simulink model "gm_sampleModel1902_sub_sub"  (R2023a)
settings: Solver=VariableStepAuto  StartTime=0.0  StopTime=10.0  RelTol=1e-3
libraries: hdlsllib x4, simulink x1
settings Model: Creator=user1  LastModifiedBy=user1
settings OptimizationCC: BlockReduction=off  ConditionallyExecuteInputs=off
settings DebuggingCC: InheritedTsInSrcMsg=none

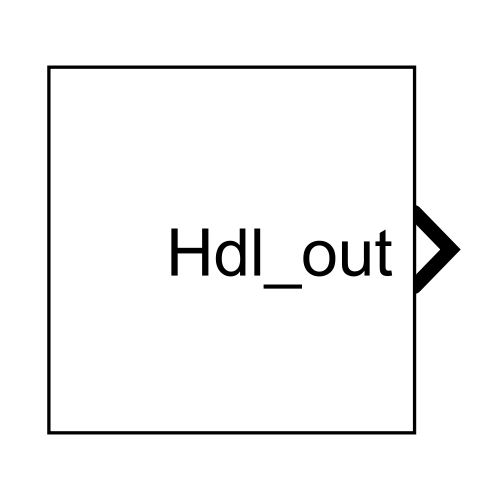
[thumbnail: Simulink's stored preview of the top-level diagram]
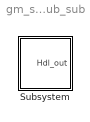
== system gm_sampleModel1902_sub_sub ==
  Subsystem : Subsystem

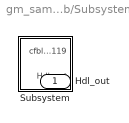
== system gm_sampleModel1902_sub_sub/Subsystem ==
  Subsystem : Subsystem
  Hdl_out : Outport  OutDataTypeStr=uint8

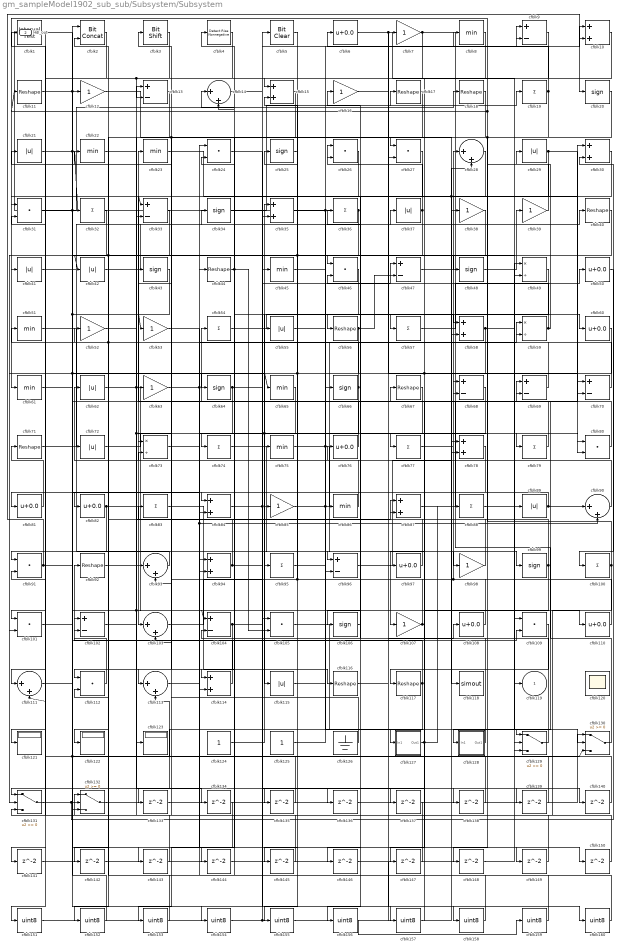
== system gm_sampleModel1902_sub_sub/Subsystem/Subsystem ==
  cfblk1 : hdlsllib/Logic and Bit Operations/Interval Test  IntervalClosedRight=on  uplimit=0.5  IntervalClosedLeft=on  lowlimit=-0.5  OutDataTypeStr=uint8
  cfblk{10,15,30,35,58,78,84,87,94,114} (10 alike) : Sum  OutDataTypeStr=uint8
  cfblk{19,32,36,54,57,74,77,79,83,88,95,100} (12 alike) : Sum  Inputs=+  OutDataTypeStr=uint8
  cfblk{24,26..27,31,46,80,91,101,105,109,112} (11 alike) : DotProduct  OutDataTypeStr=uint8
  cfblk{9,13,33,47,68..70,96,102,104} (10 alike) : Sum  Inputs=+-  OutDataTypeStr=uint8
  cfblk{14,28,90,93,103,111,113} (7 alike) : Sum  Inputs=|++  OutDataTypeStr=uint8
  cfblk{20,25,34,43,48,64,66,99,106} (9 alike) : Signum
  cfblk{7,12,16,38..39,52..53,63,85,98,107} (11 alike) : Gain  OutDataTypeStr=uint8
  cfblk{6,50,60,76,81..82,97,108,110} (9 alike) : Bias  Bias=0.0  SaturateOnIntegerOverflow=off
  cfblk{11,17..18,40,44,56,67,71,92,116..117} (11 alike) : Reshape
  cfblk{21,29,37,41..42,55,62,72,89,115} (10 alike) : Abs  OutDataTypeStr=uint8  SaturateOnIntegerOverflow=off
  cfblk118 : ToWorkspace  VariableName=simout  SaveFormat=Timeseries  SampleTime=-1
  cfblk120 : Scope
      settings: Floating=on
  cfblk121 : Display
  cfblk122 : Display
  cfblk123 : Display
  cfblk124 : Constant  OutDataTypeStr=uint8  SampleTime=-1
  cfblk125 : Constant  OutDataTypeStr=uint8  SampleTime=-1
  cfblk126 : Ground
  cfblk127 : Subsystem
      settings: LibrarySourceBlock=|
      | hdlsllib/Ports &
      | Subsystems/Subsystem
  cfblk128 : Subsystem
      settings: LibrarySourceBlock=|
      | hdlsllib/Ports &
      | Subsystems/Subsystem
  cfblk{129..132} (4 alike) : Switch  OutDataTypeStr=uint8  SaturateOnIntegerOverflow=off  InputSameDT=off
  cfblk{133..150} (18 alike) : Delay  SampleTime=1
  cfblk{151..160} (10 alike) : DataTypeConversion  OutDataTypeStr=uint8  SaturateOnIntegerOverflow=off  RndMeth=Floor
  cfblk2 : hdlsllib/Logic and Bit Operations/Bit Concat  numInputs=2
  cfblk{8,22..23,45,51,61,65,75,86} (9 alike) : MinMax  OutDataTypeStr=uint8
  cfblk3 : hdlsllib/Logic and Bit Operations/Bit Shift  mode=Shift Left Logical  N=0
  cfblk4 : hdlsllib/Logic and Bit Operations/Detect Rise Nonnegative  vinit=0  OutDataTypeStr=uint8
  cfblk49 : Product  Inputs=*/  OutDataTypeStr=uint8  RndMeth=Zero  SaturateOnIntegerOverflow=on
  cfblk5 : simulink/Logic and Bit Operations/Bit Clear  iBit=0
      settings: LibrarySourceBlock=|
      | hdlsllib/Logic and Bit
      | Operations/Bit Clear
  cfblk59 : Product  Inputs=*/  OutDataTypeStr=uint8  RndMeth=Zero  SaturateOnIntegerOverflow=on
  cfblk73 : Product  Inputs=*/  OutDataTypeStr=uint8  RndMeth=Zero  SaturateOnIntegerOverflow=on
  cfblk119 : Outport  OutDataTypeStr=uint8  VectorParamsAs1DForOutWhenUnconnected=off
  Hdl_out : Outport  Port=2  OutDataTypeStr=uint8
  wires:
  cfblk112/1 -> cfblk92/1
  cfblk51/1 -> cfblk99/1
  cfblk34/1 -> cfblk17/1
  cfblk41/1 -> cfblk34/1
  cfblk7/1 -> cfblk31/1, cfblk128/1(In1)
  cfblk105/1 -> cfblk127/1(In1)
  cfblk40/1 -> cfblk46/1
  cfblk71/1 -> cfblk40/1
  cfblk77/1 -> cfblk28/1
  cfblk124/1 -> cfblk35/1
  cfblk15/1 -> cfblk74/1
  cfblk99/1 -> cfblk16/1, cfblk131/1
  cfblk19/1 -> cfblk61/1, cfblk148/1, cfblk78/2
  cfblk86/1 -> cfblk62/1
  cfblk109/1 -> cfblk117/1
  cfblk60/1 -> cfblk97/1, cfblk82/1
  cfblk59/1 -> cfblk29/1, cfblk26/1
  cfblk65/1 -> cfblk144/1, cfblk115/1
  cfblk79/1 -> cfblk14/1
  cfblk23/1 -> cfblk70/1
  cfblk113/1 -> cfblk90/2, cfblk44/1
  cfblk46/1 -> cfblk114/1
  cfblk74/1 -> cfblk96/1
  cfblk116/1 -> cfblk108/1
  cfblk76/1 -> cfblk23/1
  cfblk73/1 -> cfblk77/1
  cfblk31/1 -> cfblk48/1, cfblk18/1
  cfblk11/1 -> cfblk143/1, cfblk12/1
  cfblk108/1 -> cfblk15/2, cfblk68/1
  cfblk129/1 -> cfblk4/1
  cfblk91/1 -> cfblk149/1, cfblk20/1
  cfblk100/1 -> cfblk8/1, cfblk132/1
  cfblk80/1 -> cfblk54/1
  cfblk97/1 -> cfblk14/2
  cfblk48/1 -> cfblk39/1
  cfblk27/1 -> cfblk103/1
  cfblk6/1 -> cfblk49/2, cfblk109/1
  cfblk54/1 -> cfblk56/1
  cfblk49/1 -> cfblk95/1
  cfblk75/1 -> cfblk10/2, cfblk107/1
  cfblk87/1 -> cfblk30/1
  cfblk33/1 -> cfblk142/1, cfblk141/1
  cfblk21/1 -> cfblk32/1, cfblk53/1, cfblk65/1, cfblk84/2
  cfblk82/1 -> cfblk132/3, cfblk98/1
  cfblk55/1 -> cfblk57/1
  cfblk42/1 -> cfblk37/1
  cfblk8/1 -> cfblk27/1
  cfblk70/1 -> cfblk3/1
  cfblk20/1 -> cfblk55/1
  cfblk44/1 -> cfblk105/2, cfblk64/1
  cfblk85/1 -> cfblk9/2, cfblk59/1
  cfblk58/1 -> cfblk130/2, cfblk122/1
  cfblk106/1 -> cfblk46/2
  cfblk29/1 -> cfblk80/1, cfblk58/2, cfblk33/1
  cfblk69/1 -> cfblk31/2, cfblk22/1
  cfblk62/1 -> cfblk96/2, cfblk119/1
  cfblk110/1 -> cfblk75/1, cfblk21/1
  cfblk32/1 -> cfblk131/2
  cfblk98/1 -> cfblk83/1
  cfblk39/1 -> cfblk11/1, cfblk6/1
  cfblk43/1 -> cfblk63/1
  cfblk57/1 -> cfblk50/1
  cfblk36/1 -> Hdl_out/1, cfblk145/1, cfblk42/1
  cfblk96/1 -> cfblk28/2
  cfblk94/1 -> cfblk139/1, cfblk72/1
  cfblk107/1 -> cfblk147/1, cfblk36/1
  cfblk78/1 -> cfblk81/1
  cfblk81/1 -> cfblk71/1
  cfblk83/1 -> cfblk116/1
  cfblk128/1(Out1) -> cfblk76/1
  cfblk68/1 -> cfblk106/1
  cfblk3/1 -> cfblk101/1
  cfblk131/1 -> cfblk30/2, cfblk130/3, cfblk109/2
  cfblk12/1 -> cfblk118/1
  cfblk22/1 -> cfblk134/1, cfblk80/2
  cfblk72/1 -> cfblk79/1
  cfblk92/1 -> cfblk93/1
  cfblk66/1 -> cfblk114/2, cfblk25/1
  cfblk88/1 -> cfblk89/1
  cfblk84/1 -> cfblk140/1, cfblk47/1
  cfblk114/1 -> cfblk102/1
  cfblk104/1 -> cfblk69/2, cfblk112/1
  cfblk89/1 -> cfblk90/1, cfblk84/1
  cfblk25/1 -> cfblk85/1
  cfblk61/1 -> cfblk110/1
  cfblk63/1 -> cfblk150/1, cfblk59/2
  cfblk17/1 -> cfblk33/2, cfblk113/1
  cfblk10/1 -> cfblk15/1
  cfblk16/1 -> cfblk70/2
  cfblk53/1 -> cfblk94/1
  cfblk125/1 -> cfblk66/1
  cfblk117/1 -> cfblk133/1, cfblk102/2
  cfblk50/1 -> cfblk100/1
  cfblk101/1 -> cfblk68/2
  cfblk95/1 -> cfblk9/1
  cfblk4/1 -> cfblk13/2, cfblk132/2
  cfblk103/1 -> cfblk45/1
  cfblk1/1 -> cfblk157/1, cfblk111/2
  cfblk30/1 -> cfblk121/1
  cfblk45/1 -> cfblk129/1
  cfblk56/1 -> cfblk47/2, cfblk135/1, cfblk101/2
  cfblk126/1 -> cfblk51/1
  cfblk127/1(Out1) -> cfblk88/1, cfblk87/1
  cfblk9/1 -> cfblk41/1
  cfblk52/1 -> cfblk104/1, cfblk123/1
  cfblk47/1 -> cfblk60/1
  cfblk37/1 -> cfblk26/2, cfblk73/1
  cfblk132/1 -> cfblk78/1
  cfblk64/1 -> cfblk138/1, cfblk94/2
  cfblk26/1 -> cfblk111/1
  cfblk102/1 -> cfblk87/2
  cfblk130/1 -> cfblk69/1
  cfblk93/1 -> cfblk91/1
  cfblk14/1 -> cfblk10/1
  cfblk35/1 -> cfblk58/1, cfblk19/1
  cfblk90/1 -> cfblk73/2
  cfblk2/1 -> cfblk151/1
  cfblk115/1 -> cfblk86/1
  cfblk133/1 -> cfblk103/2
  cfblk135/1 -> cfblk93/2
  cfblk28/1 -> cfblk136/1
  cfblk136/1 -> cfblk130/1
  cfblk18/1 -> cfblk137/1
  cfblk137/1 -> cfblk131/3
  cfblk138/1 -> cfblk113/2
  cfblk139/1 -> cfblk91/2
  cfblk140/1 -> cfblk105/1
  cfblk141/1 -> cfblk49/1
  cfblk142/1 -> cfblk129/2
  cfblk143/1 -> cfblk112/2
  cfblk144/1 -> cfblk27/2
  cfblk145/1 -> cfblk1/1
  cfblk38/1 -> cfblk146/1
  cfblk147/1 -> cfblk13/1
  cfblk148/1 -> cfblk129/3
  cfblk149/1 -> cfblk104/2
  cfblk150/1 -> cfblk43/1
  cfblk151/1 -> cfblk35/2, cfblk7/1
  cfblk13/1 -> cfblk152/1
  cfblk152/1 -> cfblk2/1
  cfblk134/1 -> cfblk153/1
  cfblk153/1 -> cfblk2/2
  cfblk111/1 -> cfblk154/1
  cfblk154/1 -> cfblk5/1
  cfblk5/1 -> cfblk155/1
  cfblk155/1 -> cfblk38/1
  cfblk67/1 -> cfblk156/1
  cfblk157/1 -> cfblk67/1
  cfblk24/1 -> cfblk158/1
  cfblk158/1 -> cfblk52/1
  cfblk156/1 -> cfblk159/1
  cfblk159/1 -> cfblk24/1
  cfblk146/1 -> cfblk160/1
  cfblk160/1 -> cfblk24/2

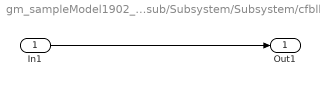
== system gm_sampleModel1902_sub_sub/Subsystem/Subsystem/cfblk127 ==
  In1 : Inport
  Out1 : Outport
  wires:
  In1/1 -> Out1/1

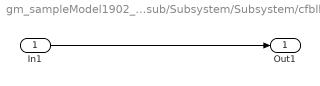
== system gm_sampleModel1902_sub_sub/Subsystem/Subsystem/cfblk128 ==
  In1 : Inport
  Out1 : Outport
  wires:
  In1/1 -> Out1/1
